simulink model "inverter_hil"  (R2024b)
settings: Solver=FixedStepDiscrete  StartTime=0.0  StopTime=inf  FixedStep=0.001  RelTol=1e-3
InitFcn:
  | enforceHardwarePreflight(bdroot);
values from neighbouring files (symbols this model uses):
  hil_cal_pedals_pressed_v1 = 1.1631952391851683    [inverter_hil.sldd]
  hil_cal_pedals_pressed_v2 = 2.341496910048066    [inverter_hil.sldd]
  hil_cal_pedals_pressed_v3 = 1.6012817578393226    [inverter_hil.sldd]
  hil_cal_pedals_pressed_v4 = 1.6012817578393226    [inverter_hil.sldd]
  hil_cal_pedals_released_v1 = 1.5156786449988555    [inverter_hil.sldd]
  hil_cal_pedals_released_v2 = 3.2025635156786452    [inverter_hil.sldd]
  hil_cal_pedals_released_v3 = 0.45445181963836118    [inverter_hil.sldd]
  hil_cal_pedals_released_v4 = 0.45445181963836118    [inverter_hil.sldd]
  hil_cmd_can_drop_control_mask = 0    [inverter_hil.sldd]
  hil_cmd_can_drop_status_mask = 0    [inverter_hil.sldd]
  hil_cmd_dc_link12_v = 0.0    [inverter_hil.sldd]
  hil_cmd_dc_link34_v = 0.0    [inverter_hil.sldd]
  hil_cmd_digital_cooling_switch = 0    [inverter_hil.sldd]
  hil_cmd_digital_main_button = 0    [inverter_hil.sldd]
  hil_cmd_digital_main_button_sequence = 0    [inverter_hil.sldd]
  hil_cmd_digital_precharge_sequence = 0    [inverter_hil.sldd]
  hil_cmd_digital_shutdown_feedback = 0    [inverter_hil.sldd]
  hil_cmd_gui_heartbeat = 0    [inverter_hil.sldd]
  hil_cmd_imu_dropout = 0    [inverter_hil.sldd]
  hil_cmd_imu_malformed = 0    [inverter_hil.sldd]
  hil_cmd_imu_stale = 0    [inverter_hil.sldd]
  hil_cmd_inverter1_connected = 1    [inverter_hil.sldd]
  hil_cmd_inverter1_fault_mask = 0    [inverter_hil.sldd]
  hil_cmd_inverter1_load_nm = 0.0    [inverter_hil.sldd]
  hil_cmd_inverter2_connected = 1    [inverter_hil.sldd]
  hil_cmd_inverter2_fault_mask = 0    [inverter_hil.sldd]
  hil_cmd_inverter2_load_nm = 0.0    [inverter_hil.sldd]
  hil_cmd_inverter3_connected = 1    [inverter_hil.sldd]
  hil_cmd_inverter3_fault_mask = 0    [inverter_hil.sldd]
  hil_cmd_inverter3_load_nm = 0.0    [inverter_hil.sldd]
  hil_cmd_inverter4_connected = 1    [inverter_hil.sldd]
  hil_cmd_inverter4_fault_mask = 0    [inverter_hil.sldd]
  hil_cmd_inverter4_load_nm = 0.0    [inverter_hil.sldd]
  hil_cmd_pedals_brake = 0.0    [inverter_hil.sldd]
  hil_cmd_pedals_plausibility_override = 0    [inverter_hil.sldd]
  hil_cmd_pedals_throttle = 0.0    [inverter_hil.sldd]
  hil_cmd_steering_angle_deg = 0.0    [inverter_hil.sldd]
  hil_cmd_steering_angle_sentinel = 0    [inverter_hil.sldd]
  hil_cmd_steering_calibration_sequence = 0    [inverter_hil.sldd]
  hil_cmd_steering_dropout = 0    [inverter_hil.sldd]
  hil_cmd_steering_invalid_status = 0    [inverter_hil.sldd]
  hil_cmd_steering_malformed = 0    [inverter_hil.sldd]
  hil_cmd_steering_speed_sentinel = 0    [inverter_hil.sldd]
  hil_cmd_steering_stale = 0    [inverter_hil.sldd]
undefined symbols (not defined in the file or in its folder): Pull, up
libraries: speedgoatlib_IO614 x21, canmsglib x16, speedgoatlib_IO183 x5
(part 3 of 3)

== matlab function inverter_hil/Hardware I O - PRE-FLIGHT DISABLED/Main Button Pulse Generator ==
  data: counter input; active output
function active = mainButtonPulseFromCounter(counter)
%MAINBUTTONPULSEFROMCOUNTER Turn a GUI counter increment into a
%fixed-width MAIN_BTN_IN pulse, mirroring
%PRECHARGEPULSEFROMCOUNTER's pulse-on-counter-change pattern: a real
%start button is pressed and released, not held. 200 ms (at the
%model's 1 ms base rate) matches the precharge pulse width.
persistent prevCounter ticksRemaining initialized
pulseTicks = uint32(200);
if isempty(initialized)
    prevCounter = counter;
    ticksRemaining = uint32(0);
    initialized = true;
end
if counter ~= prevCounter
    ticksRemaining = pulseTicks;
    prevCounter = counter;
end
%Emitted as double because that is what the IO183 Digital Output
%port takes.
active = double(ticksRemaining > uint32(0));
if ticksRemaining > uint32(0)
    ticksRemaining = ticksRemaining - uint32(1);
end
end

== matlab function inverter_hil/Ephorus System Status/CarMaker Pedal Retention ==
  data: rxDataPresent input; pedalDemand output; rxId input; rxExtended input; rxRemote input; rxLength input; rxData input
function pedalDemand = carMakerPedalRetentionStep( ...
    rxDataPresent, rxId, rxExtended, rxRemote, rxLength, rxData)
%#codegen
%CARMAKERPEDALRETENTIONSTEP One channel-1 FIFO pop per 1 ms call,
%retained and freshness-checked. See BUILD_INVERTER_HIL_MODEL's
%CARMAKERPEDALRETENTIONSCRIPT.
persistent pedalBank tickMs
if isempty(pedalBank)
    pedalBank = initialPedalDemandBank();
    tickMs = uint32(0);
end
payload = uint8(rxData(:))';
frame = struct( ...
    'id', uint32(rxId), ...
    'dlc', uint8(rxLength), ...
    'payload', payload, ...
    'isExtended', logical(rxExtended), ...
    'isRemote', logical(rxRemote), ...
    'drop', ~logical(rxDataPresent));
pedalBank = receivePedalDemandFrame(pedalBank, frame, tickMs);
pedalSnapshot = pedalDemandSnapshot(pedalBank, tickMs);
% [percent throttle, percent brake, atomic CAN ownership].
% On loss the selector returns to GUI; the GUI immediately writes zero
% on its observed handover, preventing stale slider pickup.
pedalDemand = [pedalSnapshot.throttlePercent pedalSnapshot.brakePercent double(pedalSnapshot.ownsPedals)];
%TICKMS advances 1 per call at this block's own 1 ms period, with the
%same rollover-safe MOD wrap RXRETENTIONSCRIPT uses.
tickMs = uint32(mod(double(tickMs) + 1, 4294967296));
end

== matlab function inverter_hil/Ephorus System Status/Ephorus RX Retention ==
  data: rxDataPresent input; rxObservationOut output; rxId input; rxExtended input; rxRemote input; rxLength input; rxData input; dropControlMask input; rawControlDiag output
function [rxObservationOut, rawControlDiag] = ephorusRxRetentionStep( ...
    rxDataPresent, rxId, rxExtended, rxRemote, rxLength, rxData, ...
    dropControlMask)
%#codegen
%EPHORUSRXRETENTIONSTEP Drain one CAN Read FIFO pop per call and
%retain it, at this block's own 1 ms rate. See BUILD_INVERTER_HIL_
%MODEL's RXRETENTIONSCRIPT for why: the VC's four control frames
%every 5 ms outran a single 5 ms FIFO pop.
%
%A frame is ALWAYS passed, with DROP set when nothing was received.
%RECEIVECONTROLFRAME rejects a dropped frame without touching the
%bank, so the array stays fixed-size for code generation instead of
%growing and shrinking. Nothing is fabricated: no data present means
%no command retained.
%
%BANK/STATUSBANK/TICKMS are persistent so retention survives across
%calls, exactly as the single combined block this was split out of
%used to carry it.
persistent bank statusBank tickMs
if isempty(bank)
    bank = initialDecoderBank();
    statusBank = initialStatusBank();
    tickMs = uint32(0);
end
%(:)' normalises the bus Data element to a 1x8 row regardless of the
%orientation Simulink propagates, matching the proven pattern in the
%IO614 CAN visibility test decoder.
payload = uint8(rxData(:))';
frame = struct( ...
    'id', uint32(rxId), ...
    'dlc', uint8(rxLength), ...
    'payload', payload, ...
    'isExtended', logical(rxExtended), ...
    'isRemote', logical(rxRemote), ...
    'drop', ~logical(rxDataPresent));
%TEMPORARY DIAGNOSTIC (2026-08-19): see INITIALDECODERBANK for why
%these counts are monotonic and bank-wide rather than one more
%polled-and-overwritten field. Counted from the RAW, pre-mask frame
%so the drop-mask tunable cannot hide a genuine wire mismatch from
%view. Remove this block once the control channels' permanent
%rejection is root-caused.
if ~frame.drop
    diagProtocol = protocol();
    if any(diagProtocol.controlIds == frame.id)
        bank.rawControlMatchCount = bank.rawControlMatchCount + uint32(1);
        bank.rawControlLastId = frame.id;
        bank.rawControlLastDlc = frame.dlc;
        bank.rawControlLastExtended = uint8(frame.isExtended);
        bank.rawControlLastRemote = uint8(frame.isRemote);
    end
end
statusBank = receiveStatusFrame(statusBank, frame, tickMs);
%The CAN control-frame drop mask (Fix 4) is applied to a COPY of the
%received frame used only for retention -- STATUSBANK above already
%saw the unmodified FRAME, so this mask cannot affect the received-
%status-frame path, only whether a control frame is retained into the
%decoder bank.
[controlFrame, maskDropped] = applyControlDropMask(frame, uint8(dropControlMask));
%TEMPORARY DIAGNOSTIC (2026-08-19): isolates the drop-mask tunable as
%a cause independent of everything downstream of it.
if maskDropped
    bank.maskForcedDropCount = bank.maskForcedDropCount + uint32(1);
end
bank = receiveControlFrame(bank, controlFrame, tickMs);
%RXOBSERVATION is taken BEFORE the tick advances, so the ages it
%reports are measured against the same tick the frame above was
%retained at. Advancing first would make a frame received this step
%appear one period old.
controlRows = rxObservation(bank, tickMs);
statusRows = statusObservation(statusBank, tickMs);
rxObservationOut = zeros(13, 14);
rxObservationOut(1:4, :) = controlRows;
rxObservationOut(5:13, 1:11) = statusRows;
%TEMPORARY DIAGNOSTIC (2026-08-19): see INITIALDECODERBANK/
%RAWCONTROLDIAGNOSTICS. Remove once root-caused.
rawControlDiag = rawControlDiagnostics(bank);
%TICKMS is REAL MILLISECONDS, advanced by 1 per call at this block's
%own 1 ms period. The MOD wrap matches DECODERSNAPSHOT's rollover-
%safe modulo arithmetic; MATLAB uint32 addition otherwise SATURATES
%(the generated C++ made that explicit: if (t + 1U < t) { t =
%MAX_uint32_T; }) and would freeze the counter at intmax rather than
%roll over, which would freeze every retained frame at age 0 forever
%and stop command timeouts from firing entirely.
tickMs = uint32(mod(double(tickMs) + 1, 4294967296));
end

== matlab function inverter_hil/Ephorus System Status/Ephorus Status Cycle ==
  data: rxObservation input; payloads output; loadNm1 input; loadNm2 input; loadNm3 input; loadNm4 input; connected1 input; connected2 input; connected3 input; connected4 input; dcLink12V input; dcLink34V input; steeringAngleDeg input; rxObservationOut output; txCount output; vehicleState output
function [payloads, rxObservationOut, txCount, vehicleState] = ...
        ephorusSystemStatusStep( ...
    rxObservation, ...
    loadNm1, loadNm2, loadNm3, loadNm4, ...
    connected1, connected2, connected3, connected4, ...
    dcLink12V, dcLink34V, steeringAngleDeg)
%#codegen
%EPHORUSSYSTEMSTATUSSTEP Advance the real, persistent-state Ephorus
%status cycle (see INVERTERHIL.STEPMODEL) and emit its nine 8-byte
%payloads, at the 5 ms status-cycle rate. Single source of truth:
%the hardware boundary reads PAYLOADS through a Goto/From pair rather
%than recomputing it.
%
%CAN retention itself now happens upstream in EPHORUS RX RETENTION,
%at that block's own 1 ms rate -- fast enough to keep up with the
%virtual VCU's five-CAN-ID, 5 ms burst, which a single 5 ms FIFO pop
%could not drain (see RXRETENTIONSCRIPT). RXOBSERVATION arrives here
%as that block's flattened 13x14 matrix, rate-transitioned down to
%this block's own 5 ms rate (see BUILD_INVERTER_HIL_MODEL's
%BUILDSYSTEMSTATUS). This block was deliberately NOT sped up to 1 ms
%itself: doing that once made the whole chain -- state machine,
%plant, and the CAN Pack/Write pair this block feeds -- run at 1 ms
%too, which collided with the CAN Write blocks' own explicit 5 ms
%rate (see ADDHARDWAREBOUNDARY's CAN Read comment and
%TESTMODELARTIFACTS' io614CanAndOrderedWritesAreExact guard).
%Splitting retention out is what lets the FIFO drain fast without
%moving the status/torque cadence off its real 5 ms hardware
%contract.
%
%Each channel's command is re-decoded here from RXOBSERVATION's own
%retained payload bytes with the SAME INVERTERHIL.DECODECONTROLFRAME
%the GUI and RXOBSERVATION already use, so this can never disagree
%with what the RX table shows.
%
%BANK persists only for COMMANDOUTOFDOMAIN, which is latched (plan:
%once set it stays set until the application restarts) and so cannot
%be re-derived from a single RXOBSERVATION snapshot; every other BANK
%field is refreshed from RXOBSERVATION below before use. TICKMS here
%is a fixed local reference, not a running clock: this block no
%longer measures command age itself -- RXOBSERVATION column 11
%already carries it, correctly measured against EPHORUS RX
%RETENTION's real 1 ms clock -- so LASTVALIDTICKMS below is set to
%make DECODERSNAPSHOT's own age formula (TICKMS - LASTVALIDTICKMS,
%mod 2^32) reproduce that exact value rather than measuring a second,
%inconsistent one.
%
%TXCOUNT is a genuine, target-measured count of status-cycle payloads
%this block has emitted -- one real per-call increment, not an
%estimate derived from elapsed host time (the CAN Write blocks'
%own driver exposes no cumulative transmit counter, so this is the
%actual count of cycles this block computed, which in normal
%operation, i.e. HIL_CMD_CAN_DROP_STATUS_MASK == 0, is exactly the
%count of frames each CAN Write actually sent). Shared across all 9
%status IDs since they are packed together every call; a caller
%wanting a genuinely independent per-ID count would need one counter
%per CAN Write's own Tx Control gate instead. Held in its own
%persistent TXCOUNTER, distinct from the TXCOUNT output variable:
%Simulink's MATLAB Function analysis could not determine output
%sizes/types for this block when a single variable was both
%persistent and a direct function output.
persistent state plantState bank txCounter vehicleStateBank
if isempty(state)
    state = initialSystemState();
    plantState = initialPlantState();
    bank = initialDecoderBank();
    txCounter = uint32(0);
    vehicleStateBank = [0 0 0 0];
end
tickMs = uint32(0);
controlIds = protocol().controlIds;
for channelIndex = 1:4
    bank.hasCommand(channelIndex) = rxObservation(channelIndex, 9) ~= 0;
    if bank.hasCommand(channelIndex)
        framePayload = uint8(rxObservation(channelIndex, 1:8));
        [~, ~, command] = decodeControlFrame( ...
            controlIds(channelIndex), uint8(8), framePayload, false, false);
        bank.commands(channelIndex) = command;
        ageMs = rxObservation(channelIndex, 11);
        bank.lastValidTickMs(channelIndex) = ...
            uint32(mod(double(tickMs) - ageMs, 4294967296));
    end
end
%EXTERNALINPUTS carries the GUI-commanded per-channel load torque, DC
%link pair voltage (dcLink12V feeds channels 1-2, dcLink34V feeds
%channels 3-4, matching ADDARCHITECTURE's dcPort = 1 + (channel > 2)
%convention), and connected flag into STEPMODEL -- see
%INVERTERHIL.DEFAULTEXTERNALINPUTS for why faultMask is left at its
%default (no consumer exists for it yet).
externalInputs = defaultExternalInputs();
externalInputs.channels(1).loadTorqueNm = double(loadNm1);
externalInputs.channels(2).loadTorqueNm = double(loadNm2);
externalInputs.channels(3).loadTorqueNm = double(loadNm3);
externalInputs.channels(4).loadTorqueNm = double(loadNm4);
externalInputs.channels(1).connected = logical(connected1);
externalInputs.channels(2).connected = logical(connected2);
externalInputs.channels(3).connected = logical(connected3);
externalInputs.channels(4).connected = logical(connected4);
externalInputs.channels(1).dcLinkV = double(dcLink12V);
externalInputs.channels(2).dcLinkV = double(dcLink12V);
externalInputs.channels(3).dcLinkV = double(dcLink34V);
externalInputs.channels(4).dcLinkV = double(dcLink34V);
%FRAMES is a single always-dropped frame: retention already happened
%upstream in EPHORUS RX RETENTION, so STEPMODEL must not retain
%anything a second time here. Its REJECTEDCOUNT/LASTREJECTCODE side
%effect on that dropped frame is therefore not this block's
%bookkeeping -- RXOBSERVATIONOUT below carries EPHORUS RX
%RETENTION's own correctly-tracked columns 13-14 straight through
%instead. Only COMMANDOUTOFDOMAIN, which STEPMODEL sets as a side
%effect of building PLANTINPUT from the freshly-decoded commands
%above, is read back from NEXTBANK.
droppedFrame = struct('id', uint32(0), 'dlc', uint8(0), ...
    'payload', zeros(1, 8, 'uint8'), 'isExtended', false, ...
    'isRemote', false, 'drop', true);
[state, plantState, cycle, ~, plantOutput, nextBank] = stepModel( ...
    state, plantState, tickMs, defaultStateConfig(), ...
    defaultCalibration(), bank, droppedFrame, ...
    externalInputs);
bank.commandOutOfDomain = nextBank.commandOutOfDomain;
%The MTi/LWS observations are sampled from the SAME PLANTOUTPUT this
%tick produced, so the sensor frames and the inverter status frames
%are observations of one vehicle rather than three unrelated signal
%generators. VEHICLESTATE leaves this block on port 4 and reaches the
%encoders through the HILSHAREDVEHICLESTATE Goto/From pair.
[vehicleStateBank, vehicleState] = stepVehicleState( ...
    vehicleStateBank, plantOutput, double(steeringAngleDeg), 0.005);
payloads = cycle.payloads;
rxObservationOut = rxObservation;
rxObservationOut(1:4, 12) = double(bank.commandOutOfDomain(:));
txCounter = uint32(mod(double(txCounter) + 1, 4294967296));
txCount = txCounter;
end

== matlab function inverter_hil/Hardware I O - PRE-FLIGHT DISABLED/Synchronized Sensor Payloads ==
  data: vehicleState input; acceleration output; steeringAngleDeg input; imuDropout input; steeringDropout input; imuStale input; steeringStale input; imuMalformed input; steeringMalformed input; invalidStatus input; angleSentinel input; speedSentinel input; calibrationSequence input; rateOfTurn output; velocity output; steering output; config output; enableAcceleration output; enableRateOfTurn output; enableVelocity output; enableSteering output; enableConfig output; txCounts output; agesS output; calibrationState output; dlcAcceleration output; dlcRateOfTurn output; dlcVelocity output; dlcSteering output; dlcConfig output
function [acceleration, rateOfTurn, velocity, steering, config, ...
    enableAcceleration, enableRateOfTurn, enableVelocity, ...
    enableSteering, enableConfig, txCounts, agesS, ...
    calibrationState, dlcAcceleration, dlcRateOfTurn, dlcVelocity, ...
    dlcSteering, dlcConfig] = synchronizedSensorPayloads( ...
    vehicleState, steeringAngleDeg, imuDropout, steeringDropout, ...
    imuStale, steeringStale, imuMalformed, steeringMalformed, ...
    invalidStatus, angleSentinel, speedSentinel, calibrationSequence)
%#codegen
%SYNCHRONIZEDSENSORPAYLOADS Encode the independent sensor contracts.
%VEHICLESTATE is the 1x9 [ax ay az wx wy wz vx vy vz] observation
%produced by
%the SAME inverter-plant tick (INVERTERHIL.STEPVEHICLESTATE's second
%output), so these frames and the Ephorus status frames describe one
%vehicle rather than three unrelated generators.
% Calibration state: 0 idle, 1 reset pending, 2 reset verification,
%3 zero pending, 4 zero verification, 5 passed, 6 failed. The 100 ms
%inter-command hold is a conservative HIL policy (ten Bosch update
%periods), not a datasheet claim. Zero is never emitted until the
%target has observed an uncalibrated 0x2B0 response after reset.
%Every output is initialized before persistent state or protocol
%helpers are touched. R2024b Stateflow analysis otherwise cannot prove
%the fixed dimensions of this 12-input/18-output chart.
%PERSISTENT MUST COME FIRST. Plain MATLAB tolerates a persistent
%declaration after executable code, but the MATLAB Function block
%does not: it rejects the whole chart with
%STATEFLOW:CDR:ERRORSPARSINGEMLFCN, which reports a parse failure
%and names no line. Keep this block above the output
%initialisation below, even though the initialisation is what makes
%the fixed output dimensions provable.
persistent phase lastSteeringDeg cachedAcceleration cachedRate ...
    cachedVelocity cachedSteering cachedConfig counters imuAgeS steeringAgeS ...
    configAgeS requestSeen calibrationPhase calibrationElapsedS ...
    simulatedCalibrated zeroOffsetDeg
acceleration = zeros(1,6,'uint8');
rateOfTurn = zeros(1,6,'uint8');
velocity = zeros(1,6,'uint8');
steering = zeros(1,5,'uint8');
config = zeros(1,2,'uint8');
enableAcceleration = uint32(0); enableRateOfTurn = uint32(0);
enableVelocity = uint32(0); enableSteering = uint32(0);
enableConfig = uint32(0);
txCounts = zeros(1,5,'uint32'); agesS = zeros(1,5);
calibrationState = uint8(0);
dlcAcceleration = uint8(6); dlcRateOfTurn = uint8(6);
dlcVelocity = uint8(6); dlcSteering = uint8(5); dlcConfig = uint8(2);
stateVector = zeros(1,9);
for stateIndex = 1:9
    stateVector(stateIndex) = double(vehicleState(stateIndex));
end
if isempty(phase)
    phase = uint8(0);
    lastSteeringDeg = double(steeringAngleDeg);
    cachedAcceleration = zeros(1,6,'uint8');
    cachedRate = zeros(1,6,'uint8');
    cachedVelocity = zeros(1,6,'uint8');
    cachedSteering = zeros(1,5,'uint8');
    cachedConfig = zeros(1,2,'uint8');
    counters = zeros(1,5,'uint32');
    imuAgeS = 0; steeringAgeS = 0; configAgeS = -1;
    requestSeen = uint32(0); calibrationPhase = uint8(0);
    calibrationElapsedS = 0; simulatedCalibrated = true;
    zeroOffsetDeg = 0;
end
angleDeg = double(steeringAngleDeg);
config = cachedConfig; enableConfig = uint32(0);
sequence = uint32(calibrationSequence);
if sequence ~= requestSeen
    requestSeen = sequence;
    if calibrationPhase == 0 || calibrationPhase >= 5
        calibrationPhase = uint8(1); calibrationElapsedS = 0;
    end
end
if calibrationPhase == 1
    config = packLwsConfigPayload(uint8(5));
    cachedConfig = config;
    enableConfig = uint32(1); simulatedCalibrated = false;
    calibrationPhase = uint8(2); calibrationElapsedS = 0;
elseif calibrationPhase == 3
    config = packLwsConfigPayload(uint8(3));
    cachedConfig = config;
    enableConfig = uint32(1); simulatedCalibrated = true;
    zeroOffsetDeg = angleDeg;
    calibrationPhase = uint8(4); calibrationElapsedS = 0;
end
if enableConfig ~= 0
    counters(5) = uint32(mod(double(counters(5)) + 1, 4294967296));
    configAgeS = 0;
elseif configAgeS >= 0
    configAgeS = configAgeS + 0.005;
end
enableAcceleration = uint32(~logical(imuDropout));
enableRateOfTurn = enableAcceleration; enableVelocity = enableAcceleration;
if enableAcceleration ~= 0
    counters(1) = uint32(mod(double(counters(1)) + 1, 4294967296));
    counters(2) = uint32(mod(double(counters(2)) + 1, 4294967296));
    counters(3) = uint32(mod(double(counters(3)) + 1, 4294967296));
end
if enableAcceleration ~= 0 && ~logical(imuStale)
    cachedAcceleration = packMti680Payload('acceleration', stateVector(1:3));
    cachedRate = packMti680Payload('rateofturn', stateVector(4:6));
    cachedVelocity = packMti680Payload('velocityxyz', stateVector(7:9));
    imuAgeS = 0;
else
    imuAgeS = imuAgeS + 0.005;
end
acceleration = cachedAcceleration; rateOfTurn = cachedRate;
velocity = cachedVelocity;
%LWS_SPEED is the STEERING WHEEL angular speed -- the Bosch datasheet
%defines it as "Angular speed", 0 to 1016 deg/s at 4 deg/s resolution,
%i.e. the rate of change of LWS_ANGLE. It is NOT the vehicle yaw rate,
%which is a different physical quantity on a different sensor (the
%MTi rate-of-turn frame above already carries yaw rate). Derived here
%from successive 10 ms LWS samples and clamped
%into the encoder range so a fast dial sweep cannot range-error
%PACKLWSPAYLOAD.
lwsDue = mod(phase, uint8(2)) == 0; lwsUpdated = false;
enableSteering = uint32(~logical(steeringDropout) && lwsDue);
if enableSteering ~= 0
    counters(4) = uint32(mod(double(counters(4)) + 1, 4294967296));
end
if enableSteering ~= 0 && ~logical(steeringStale)
    speedDegPerS = min(1016, abs(angleDeg - lastSteeringDeg) / 0.010);
    lastSteeringDeg = angleDeg;
    reportedAngleDeg = min(780, max(-780, angleDeg - zeroOffsetDeg));
    candidate = zeros(1,5,'uint8');
    candidate = packLwsPayload(reportedAngleDeg, speedDegPerS, uint8(7));
    if ~simulatedCalibrated
        candidate(1) = uint8(255); candidate(2) = uint8(127);
        candidate(4) = uint8(5);
    end
    if logical(invalidStatus); candidate(4) = uint8(2); end
    if logical(angleSentinel)
        candidate(1) = uint8(255); candidate(2) = uint8(127);
    end
    if logical(speedSentinel); candidate(3) = uint8(255); end
    cachedSteering = candidate; steeringAgeS = 0; lwsUpdated = true;
else
    steeringAgeS = steeringAgeS + 0.005;
end
steering = cachedSteering;
%The LWS updates at 100 Hz / 10 ms (datasheet "CAN update rate") and
%this block runs at the 5 ms status rate, so every second tick
%transmits. A dropout is a genuine absence on the wire (Tx Control
%low), not a zeroed payload.
if calibrationPhase == 2
    calibrationElapsedS = calibrationElapsedS + 0.005;
    if calibrationElapsedS >= 0.100
        resetObserved = cachedSteering(1) == 255 && ...
            cachedSteering(2) == 127 && cachedSteering(3) ~= 255 && ...
            cachedSteering(4) == 5;
        if resetObserved
            calibrationPhase = uint8(3);
        else
            calibrationPhase = uint8(6);
        end
    end
elseif calibrationPhase == 4
    calibrationElapsedS = calibrationElapsedS + 0.005;
    if calibrationElapsedS >= 0.010 && lwsUpdated
        zeroObserved = cachedSteering(1) == 0 && ...
            cachedSteering(2) == 0 && cachedSteering(3) ~= 255 && ...
            cachedSteering(4) == 7;
        if zeroObserved
            calibrationPhase = uint8(5);
        else
            calibrationPhase = uint8(6);
        end
    elseif calibrationElapsedS >= 0.100
        calibrationPhase = uint8(6);
    end
end
phase = uint8(mod(double(phase) + 1, 2));
txCounts = counters;
agesS = [imuAgeS imuAgeS imuAgeS steeringAgeS configAgeS];
calibrationState = calibrationPhase;
if logical(imuMalformed)
    dlcAcceleration = uint8(5); dlcRateOfTurn = uint8(5);
    dlcVelocity = uint8(5);
end
if logical(steeringMalformed); dlcSteering = uint8(4); end
end
